simulink model "jifenfenli"  (R2022a)
settings: Solver=FixedStepAuto  StartTime=0.0  StopTime=1  RelTol=1e-3
values from neighbouring files (symbols this model uses):
  ki = 0.01    [karina.m]
  kp = 0.20    (= 0.2)    [karina.m]
undefined symbols (not defined in the file or in its folder): den, denQ, DiscIntNeverNeededParam, num, numQ
settings Model: Creator=Userx  LastModifiedBy=Userx

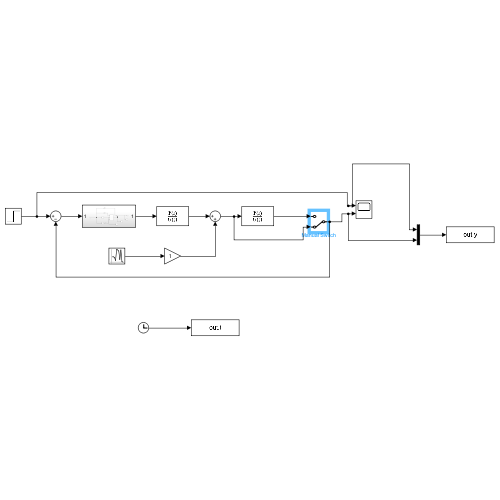
[thumbnail: Simulink's stored preview of the top-level diagram]
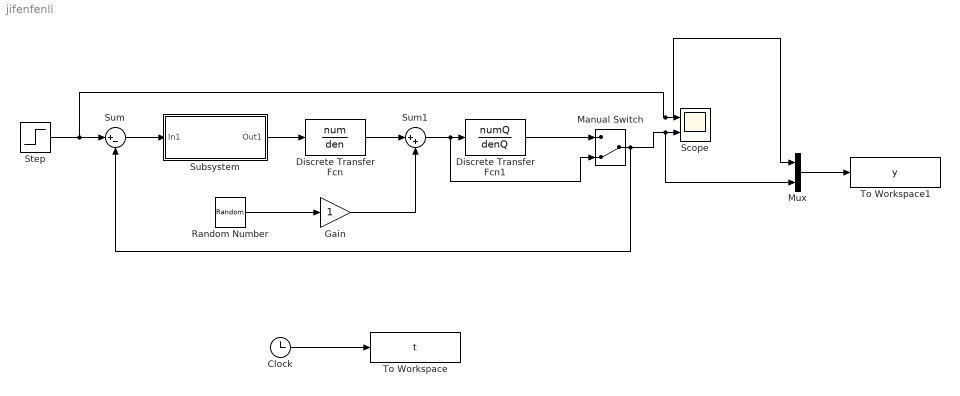
== system jifenfenli ==
  Clock : Clock
  Discrete Transfer Fcn : DiscreteTransferFcn  Numerator=num  Denominator=den
  Discrete Transfer Fcn1 : DiscreteTransferFcn  Numerator=numQ  Denominator=denQ
  Gain : Gain
  Manual Switch : ManualSwitch  CurrentSetting=0
  Mux : Mux  Inputs=2
  Random Number : RandomNumber  Variance=8.33  SampleTime=0.001
  Scope : Scope  NumInputPorts=2
  Step : Step  Time=0  After=20  SampleTime=0.001
  Subsystem : Subsystem
  Sum : Sum  Inputs=|+-
  Sum1 : Sum  Inputs=|++
  To Workspace : ToWorkspace  VariableName=t  SampleTime=-1
  To Workspace1 : ToWorkspace  VariableName=y  SampleTime=-1
  wires:
  Step/1 -> Mux/1, Scope/1, Sum/1
  Sum/1 -> Subsystem/1(In1)
  Clock/1 -> To Workspace/1
  Subsystem/1(Out1) -> Discrete Transfer Fcn/1
  Random Number/1 -> Gain/1
  Gain/1 -> Sum1/2
  Discrete Transfer Fcn/1 -> Sum1/1
  Sum1/1 -> Manual Switch/2, Discrete Transfer Fcn1/1
  Discrete Transfer Fcn1/1 -> Manual Switch/1
  Manual Switch/1 -> Sum/2, Mux/2, Scope/2
  Mux/1 -> To Workspace1/1

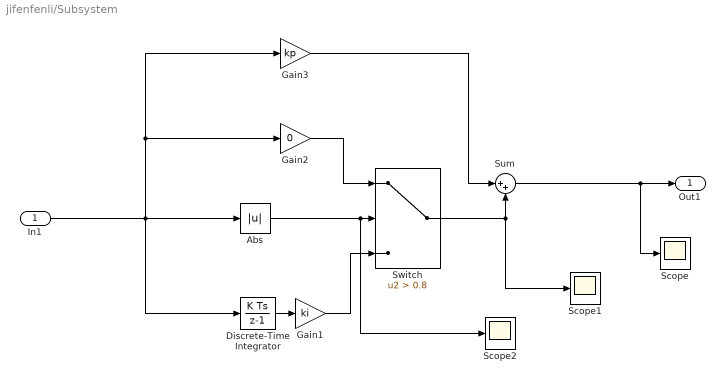
== system jifenfenli/Subsystem ==
  In1 : Inport
  Abs : Abs  SaturateOnIntegerOverflow=off
  Discrete-Time Integrator : DiscreteIntegrator  SampleTime=-1  ICPrevOutput=DiscIntNeverNeededParam  ICPrevScaledInput=DiscIntNeverNeededParam
  Gain1 : Gain  Gain=ki
  Gain2 : Gain  Gain=0
  Gain3 : Gain  Gain=kp
  Scope : Scope
  Scope1 : Scope
  Scope2 : Scope
  Sum : Sum  Inputs=|++
  Switch : Switch  Criteria=u2 > Threshold  Threshold=0.8  SaturateOnIntegerOverflow=off  InputSameDT=off
  Out1 : Outport
  wires:
  Abs/1 -> Scope2/1, Switch/2
  Discrete-Time Integrator/1 -> Gain1/1
  In1/1 -> Discrete-Time Integrator/1, Abs/1, Gain2/1, Gain3/1
  Gain1/1 -> Switch/3
  Gain2/1 -> Switch/1
  Gain3/1 -> Sum/1
  Switch/1 -> Scope1/1, Sum/2
  Sum/1 -> Scope/1, Out1/1
